simulink model "BBBC_6"  (R2022b)
settings: Solver=VariableStepAuto  StartTime=0.0  StopTime=5  RelTol=1e-3
undefined symbols (not defined in the file): dct, dEv, Ev, sigbuilder_block
libraries: spsMosfetLib x4, spsSeriesRLCBranchLib x4, spsCurrentMeasurementLib x2, spsVoltageMeasurementLib x2, spsGroundLib x1, spsControlledVoltageSourceLib x1, simulink x1, spspowerguiLib x1
settings Model: Creator=Dopechuro  LastModifiedBy=Dopechuro

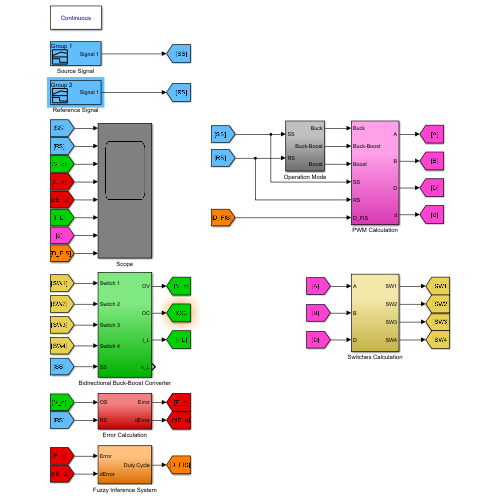
[thumbnail: Simulink's stored preview of the top-level diagram]
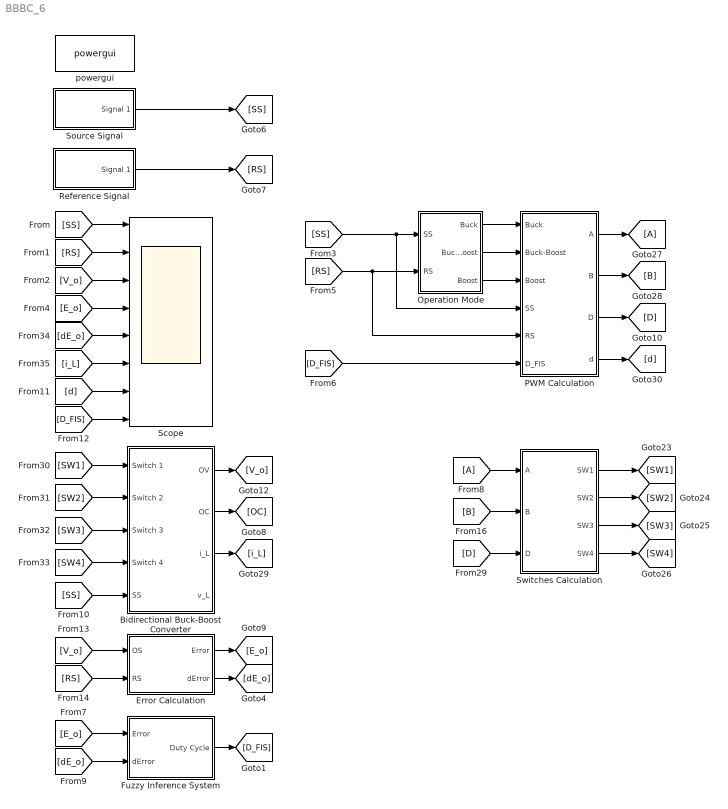
== system BBBC_6 ==
  Bidirectional Buck-Boost Converter : Subsystem
  Error Calculation : Subsystem
  From8 : From
  Fuzzy Inference System : Subsystem
  Goto27 : Goto
  Operation Mode : Subsystem
  PWM Calculation : Subsystem
  Reference Signal : Subsystem  Tag=STV Subsys  LoadFcn=sigbuilder_block('load');  StartFcn=sigbuilder_block('start');  StopFcn=sigbuilder_block('stop');  ClipboardFcn=sigbuilder_block('clipboard');  mask(Sigbuilder block){tuvar=[0:10]}
      mask help: Simulink:masks:SigbuilderBlock_MD
      mask init:
      | if ~strcmp(get_param(bdroot(gcbh),'SimulationStatus'),'stopped') tuvar = sigbuilder_block('maskInit'); end
      settings: CopyFcn=sigbuilder_block('copy');  DeleteFcn=sigbuilder_block('delete');  ModelCloseFcn=sigbuilder_block('modelClose');  PreSaveFcn=sigbuilder_block('preSave');  PauseFcn=sigbuilder_block('pause');  ContinueFcn=sigbuilder_block('continue');  NameChangeFcn=sigbuilder_block('namechange');  OpenFcn=sigbuilder_block('open',[530.25 309.75 550.5 399.75 ]);  CloseFcn=sigbuilder_block('close');
      mask Display: plot(0, 0, 100, 100,[2, 2, 32, 32, 2], [68, 8, 8, 68, 68],[32, 2], [38, 38], [32, 19, 2],[53, 60, 44], [32, 17, 17, 2],[16, 16, 31, 31]);txt = getActiveGroup(gcbh);text(2, 100, txt,'verticalAlignment', 'top');
  Scope : Scope  NumInputPorts=8
  Source Signal : Subsystem  Tag=STV Subsys  LoadFcn=sigbuilder_block('load');  StartFcn=sigbuilder_block('start');  StopFcn=sigbuilder_block('stop');  ClipboardFcn=sigbuilder_block('clipboard');  mask(Sigbuilder block){tuvar=[0:10]}
      mask help: Simulink:masks:SigbuilderBlock_MD
      mask init:
      | if ~strcmp(get_param(bdroot(gcbh),'SimulationStatus'),'stopped') tuvar = sigbuilder_block('maskInit'); end
      settings: CopyFcn=sigbuilder_block('copy');  DeleteFcn=sigbuilder_block('delete');  ModelCloseFcn=sigbuilder_block('modelClose');  PreSaveFcn=sigbuilder_block('preSave');  PauseFcn=sigbuilder_block('pause');  ContinueFcn=sigbuilder_block('continue');  NameChangeFcn=sigbuilder_block('namechange');  OpenFcn=sigbuilder_block('open',[325.5 242.25 550.5 399.75 ]);  CloseFcn=sigbuilder_block('close');
      mask Display: plot(0, 0, 100, 100,[2, 2, 32, 32, 2], [68, 8, 8, 68, 68],[32, 2], [38, 38], [32, 19, 2],[53, 60, 44], [32, 17, 17, 2],[16, 16, 31, 31]);txt = getActiveGroup(gcbh);text(2, 100, txt,'verticalAlignment', 'top');
  Switches Calculation : Subsystem
  powergui : spspowerguiLib/powergui  Priority=1  SimulationMode=Continuous  SampleTime=50e-6  frequency=60  Iterations=50  frequencyindice=0  Pbase=100e6  ErrMax=1e-4  UnitsV=kV  UnitsW=MW  buscounter=0  FunctionMessages=off  echomessages=off  EnableUseOfTLC=off  CurrentSourceSwitches=off  DisableSnubberDevices=off  DisableRonSwitches=off  DisableVfSwitches=off  DisplayEquations=off  AutomaticDiscreteSolvers=off  SolverType=Tustin/Backward Euler (TBE)  Interpol=off  ExternalGateDelay=off  methode=off  Ts=100  x0status=blocks  SPID=on  SwTol=0  HookPort=off  NonlinearTolerance=1e-4  nMaxIteration=100  ContinueOnMaxIteration=off  RestoreLinks=warning  ResistiveCurrentMeasurement=off  Frange=[0:2:500]  Ylog=off  Xlog=on  ShowGrid=off  save=off  variable=ZData  structure=0  ZoomFFT=off  StartTime=0.0  cycles=1  DisplayStyle=1  fundamental=60  FreqAxis=off  MaxFrequency=1000  frequencyindicesteady=1  RmsSteady=1  display=off
  wires:
  [RS] -> Scope/2
  [V_o] -> Scope/3
  [V_o] -> Error Calculation/1(OS)
  [RS] -> Error Calculation/2(RS)
  Error Calculation/1(Error) -> [E_o]
  Error Calculation/2(dError) -> [dE_o]
  [SS] -> Scope/1
  [SS] -> Bidirectional Buck-Boost Converter/5(SS)
  Bidirectional Buck-Boost Converter/1(OV) -> [V_o]
  [E_o] -> Fuzzy Inference System/1(Error)
  [dE_o] -> Fuzzy Inference System/2(dError)
  Fuzzy Inference System/1(Duty Cycle) -> [D_FIS]
  Bidirectional Buck-Boost Converter/2(OC) -> [OC]
  [E_o] -> Scope/4
  [SW1] -> Bidirectional Buck-Boost Converter/1(Switch 1)
  [SW2] -> Bidirectional Buck-Boost Converter/2(Switch 2)
  [SW3] -> Bidirectional Buck-Boost Converter/3(Switch 3)
  [SW4] -> Bidirectional Buck-Boost Converter/4(Switch 4)
  Source Signal/1(Signal 1) -> [SS]
  Reference Signal/1(Signal 1) -> [RS]
  Bidirectional Buck-Boost Converter/3(i_L) -> [i_L]
  [dE_o] -> Scope/5
  [i_L] -> Scope/6
  From8/1 -> Switches Calculation/1(A)
  [B] -> Switches Calculation/2(B)
  [D] -> Switches Calculation/3(D)
  Switches Calculation/1(SW1) -> [SW1]
  Switches Calculation/2(SW2) -> [SW2]
  Switches Calculation/3(SW3) -> [SW3]
  Switches Calculation/4(SW4) -> [SW4]
  [RS] -> Operation Mode/2(RS), PWM Calculation/5(RS)
  Operation Mode/1(Buck) -> PWM Calculation/1(Buck)
  Operation Mode/2(Buck-Boost) -> PWM Calculation/2(Buck-Boost)
  Operation Mode/3(Boost) -> PWM Calculation/3(Boost)
  [D_FIS] -> PWM Calculation/6(D_FIS)
  PWM Calculation/3(D) -> [D]
  PWM Calculation/4(d) -> [d]
  PWM Calculation/1(A) -> Goto27/1
  PWM Calculation/2(B) -> [B]
  [d] -> Scope/7
  [D_FIS] -> Scope/8
  [SS] -> PWM Calculation/4(SS), Operation Mode/1(SS)

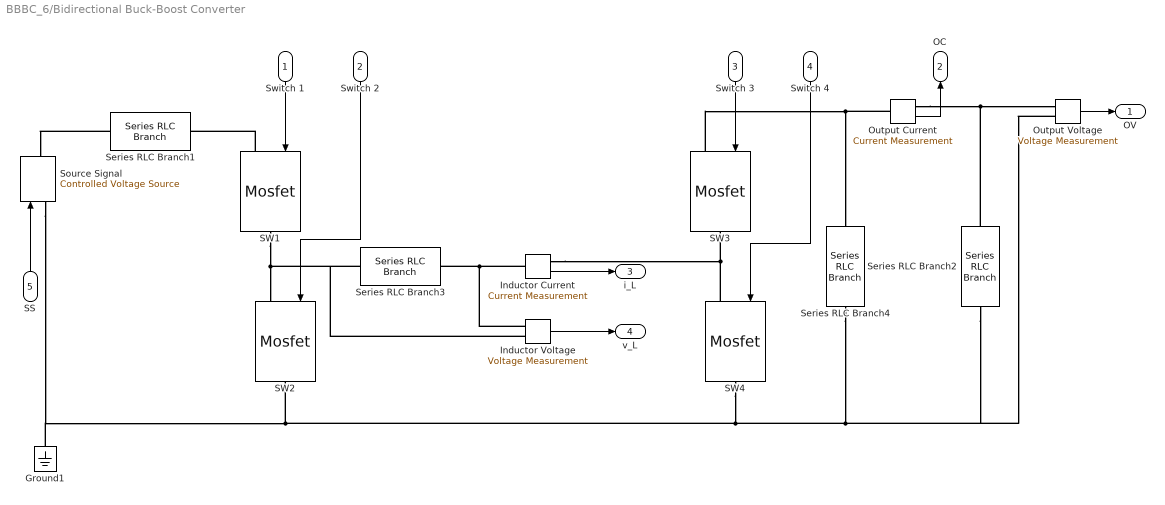
== system BBBC_6/Bidirectional Buck-Boost Converter ==
  Switch 1 : Inport
  Switch 2 : Inport  Port=2
  Switch 3 : Inport  Port=3
  Switch 4 : Inport  Port=4
  SS : Inport  Port=5
  Ground1 : spsGroundLib/Ground  LConnTagsString=a
  Inductor Current : spsCurrentMeasurementLib/Current Measurement  PhasorSimulation=off  OutputType=Complex  PSBequivalent=0
  Inductor Voltage : spsVoltageMeasurementLib/Voltage Measurement  PhasorSimulation=off  OutputType=Complex  PSBequivalent=0
  Output Current : spsCurrentMeasurementLib/Current Measurement  PhasorSimulation=off  OutputType=Complex  PSBequivalent=0
  Output Voltage : spsVoltageMeasurementLib/Voltage Measurement  PhasorSimulation=off  OutputType=Complex  PSBequivalent=0
  SW{1..4} (4 alike) : spsMosfetLib/Mosfet  Ron=0.1  Lon=0  Rd=0.01  Vfd=0  IC=0  Rs=1e5  Cs=inf  Measurements=off
  Series RLC Branch1 : spsSeriesRLCBranchLib/Series RLC Branch  LConnTagsString=__new0  RConnTagsString=__new0  BranchType=R  Resistance=0.1  Inductance=1e-3  SetiL0=off  InitialCurrent=0  Capacitance=1e-6  Setx0=off  InitialVoltage=0  Measurements=None
  Series RLC Branch2 : spsSeriesRLCBranchLib/Series RLC Branch  LConnTagsString=__new0  RConnTagsString=__new0  BranchType=R  Resistance=24  Inductance=1e-3  SetiL0=off  InitialCurrent=0  Capacitance=1000e-6  Setx0=off  InitialVoltage=0  Measurements=None
  Series RLC Branch3 : spsSeriesRLCBranchLib/Series RLC Branch  LConnTagsString=__new0  RConnTagsString=__new0  BranchType=RL  Resistance=0.1  Inductance=0.434e-3  SetiL0=off  InitialCurrent=0  Capacitance=1e-6  Setx0=off  InitialVoltage=0  Measurements=None
  Series RLC Branch4 : spsSeriesRLCBranchLib/Series RLC Branch  LConnTagsString=__new0  RConnTagsString=__new0  BranchType=RC  Resistance=0.01  Inductance=1e-3  SetiL0=off  InitialCurrent=0  Capacitance=10.6e-6  Setx0=off  InitialVoltage=0  Measurements=None
  Source Signal : spsControlledVoltageSourceLib/Controlled Voltage Source  Initialize=off  Source_Type=DC  Amplitude=0  Phase=0  Frequency=0  Measurements=None
  OV : Outport
  OC : Outport  Port=2
  i_L : Outport  Port=3
  v_L : Outport  Port=4
  wires:
  Switch 1/1 -> SW1/1
  Switch 3/1 -> SW3/1
  Switch 2/1 -> SW2/1
  SS/1 -> Source Signal/1
  Switch 4/1 -> SW4/1
  Inductor Current/1 -> i_L/1
  Output Voltage/1 -> OV/1
  Inductor Voltage/1 -> v_L/1
  Output Current/1 -> OC/1
  connections:
  SW1/LConn1 -- Series RLC Branch1/RConn1
  Inductor Current/LConn1 -- Inductor Voltage/LConn2 -- Series RLC Branch3/RConn1
  SW4/LConn1 -- Inductor Current/RConn1 -- SW3/RConn1
  SW4/RConn1 -- Output Voltage/LConn2 -- Series RLC Branch2/RConn1 -- Series RLC Branch4/RConn1 -- Source Signal/LConn1 -- Ground1/LConn1 -- SW2/RConn1
  SW1/RConn1 -- Inductor Voltage/LConn1 -- Series RLC Branch3/LConn1 -- SW2/LConn1
  Series RLC Branch1/LConn1 -- Source Signal/RConn1
  Output Current/RConn1 -- Output Voltage/LConn1 -- Series RLC Branch2/LConn1
  SW3/LConn1 -- Output Current/LConn1 -- Series RLC Branch4/LConn1

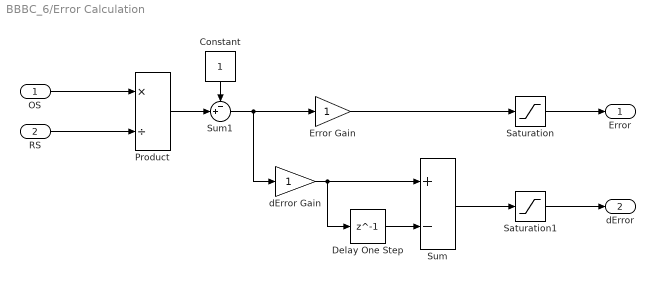
== system BBBC_6/Error Calculation ==
  OS : Inport
  RS : Inport  Port=2
  Constant : Constant
  Delay One Step : Delay  DelayLength=1
  Error Gain : Gain
  Product : Product  Inputs=*/
  Saturation : Saturate  UpperLimit=1  LowerLimit=-1
  Saturation1 : Saturate  UpperLimit=1  LowerLimit=-1
  Sum : Sum  Inputs=+-
  Sum1 : Sum  Inputs=-+|
  dError Gain : Gain
  Error : Outport
  dError : Outport  Port=2
  wires:
  Sum1/1 -> dError Gain/1, Error Gain/1
  dError Gain/1 -> Sum/1, Delay One Step/1
  Error Gain/1 -> Saturation/1
  Constant/1 -> Sum1/1
  Delay One Step/1 -> Sum/2
  Product/1 -> Sum1/2
  Sum/1 -> Saturation1/1
  OS/1 -> Product/1
  RS/1 -> Product/2
  Saturation/1 -> Error/1
  Saturation1/1 -> dError/1

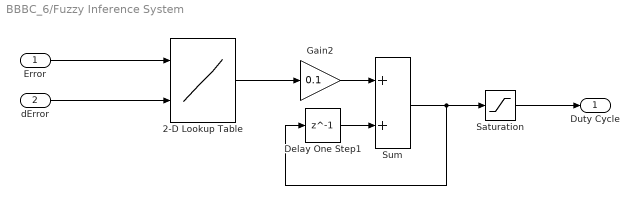
== system BBBC_6/Fuzzy Inference System ==
  Error : Inport
  dError : Inport  Port=2
  2-D Lookup Table : Lookup_n-D  LookupTableObject=''  BreakpointsForDimension1=Ev  BreakpointsForDimension2=dEv  BreakpointsForDimension1FirstPoint=10  BreakpointsForDimension2FirstPoint=10  BreakpointsForDimension1Spacing=12  BreakpointsForDimension2Spacing=12  IndexSearchMethod=Evenly spaced points  Table=dct  InterpMethod=Nearest  DiagnosticForOutOfRangeInput=Warning  InternalRulePriority=Speed  OutDataTypeStr=Inherit: Inherit from 'Table data'  RndMeth=Simplest
      settings: InputPortMap=u0,u1
  Delay One Step1 : Delay  DelayLength=1
  Gain2 : Gain  Gain=0.1
  Saturation : Saturate  UpperLimit=0.9  LowerLimit=-0.9
  Sum : Sum
  Duty Cycle : Outport
  wires:
  Delay One Step1/1 -> Sum/2
  Sum/1 -> Saturation/1, Delay One Step1/1
  Gain2/1 -> Sum/1
  2-D Lookup Table/1 -> Gain2/1
  Saturation/1 -> Duty Cycle/1
  Error/1 -> 2-D Lookup Table/1
  dError/1 -> 2-D Lookup Table/2

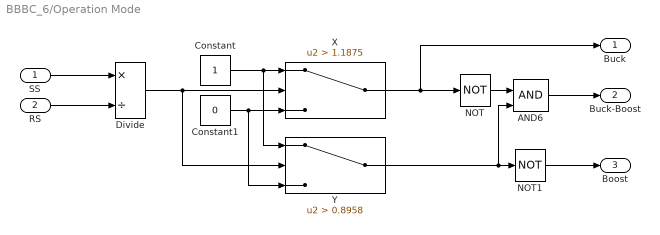
== system BBBC_6/Operation Mode ==
  SS : Inport
  RS : Inport  Port=2
  AND6 : Logic  IconShape=distinctive  AllPortsSameDT=off  OutDataTypeStr=boolean
  Constant : Constant
  Constant1 : Constant  Value=0
  Divide : Product  Inputs=*/
  NOT : Logic  Operator=NOT  IconShape=distinctive  AllPortsSameDT=off  OutDataTypeStr=boolean
  NOT1 : Logic  Operator=NOT  IconShape=distinctive  AllPortsSameDT=off  OutDataTypeStr=boolean
  X : Switch  Criteria=u2 > Threshold  Threshold=1.1875  SaturateOnIntegerOverflow=off  InputSameDT=off
  Y : Switch  Criteria=u2 > Threshold  Threshold=0.8958  SaturateOnIntegerOverflow=off  InputSameDT=off
  Buck : Outport
  Buck-Boost : Outport  Port=2
  Boost : Outport  Port=3
  wires:
  RS/1 -> Divide/2
  Constant/1 -> Y/1, X/1
  Divide/1 -> Y/2, X/2
  X/1 -> Buck/1, NOT/1
  NOT/1 -> AND6/1
  Constant1/1 -> Y/3, X/3
  Y/1 -> NOT1/1, AND6/2
  SS/1 -> Divide/1
  AND6/1 -> Buck-Boost/1
  NOT1/1 -> Boost/1

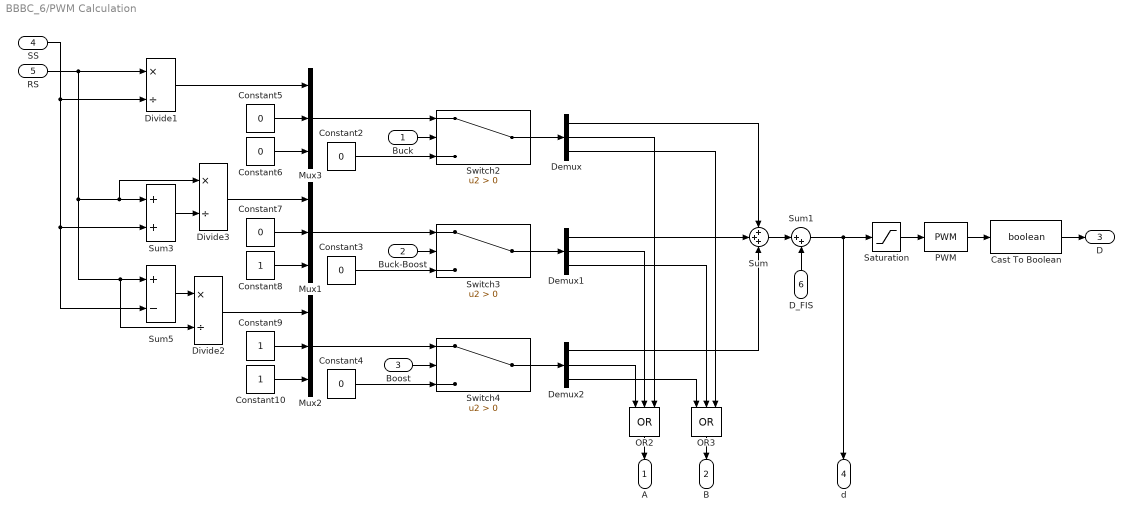
== system BBBC_6/PWM Calculation ==
  Buck : Inport
  Buck-Boost : Inport  Port=2
  Boost : Inport  Port=3
  SS : Inport  Port=4
  RS : Inport  Port=5
  D_FIS : Inport  Port=6
  Cast To Boolean : DataTypeConversion  OutDataTypeStr=boolean  SaturateOnIntegerOverflow=off  RndMeth=Floor
  Constant10 : Constant
  Constant{2..7} (6 alike) : Constant  Value=0
  Constant8 : Constant
  Constant9 : Constant
  Demux : Demux  Outputs=3
  Demux1 : Demux  Outputs=3
  Demux2 : Demux  Outputs=3
  Divide1 : Product  Inputs=*/
  Divide2 : Product  Inputs=*/
  Divide3 : Product  Inputs=*/
  Mux1 : Mux  Inputs=3
  Mux2 : Mux  Inputs=3
  Mux3 : Mux  Inputs=3
  OR2 : Logic  Operator=OR  Inputs=3  IconShape=distinctive  AllPortsSameDT=off  OutDataTypeStr=boolean
  OR3 : Logic  Operator=OR  Inputs=3  IconShape=distinctive  AllPortsSameDT=off  OutDataTypeStr=boolean
  PWM : simulink/Discontinuities/PWM  DisableCoverage=on  Period=1e-5  InitialDelay=0  DisallowZeroDutyCycle=off  RunAtFixedTimeIntervals=off  SampleTime=0.1
  Saturation : Saturate  UpperLimit=0.85  LowerLimit=0.1
  Sum : Sum  Inputs=+++
  Sum1 : Sum  Inputs=|++
  Sum3 : Sum
  Sum5 : Sum  Inputs=+-
  Switch2 : Switch  Criteria=u2 > Threshold  SaturateOnIntegerOverflow=off  InputSameDT=off
  Switch3 : Switch  Criteria=u2 > Threshold  SaturateOnIntegerOverflow=off  InputSameDT=off
  Switch4 : Switch  Criteria=u2 > Threshold  SaturateOnIntegerOverflow=off  InputSameDT=off
  A : Outport
  B : Outport  Port=2
  D : Outport  Port=3
  d : Outport  Port=4
  wires:
  Constant6/1 -> Mux3/3
  Constant2/1 -> Switch2/3
  Switch4/1 -> Demux2/1
  Sum3/1 -> Divide3/2
  Constant5/1 -> Mux3/2
  Mux3/1 -> Switch2/1
  Sum1/1 -> Saturation/1, d/1
  Constant8/1 -> Mux1/3
  Demux1/1 -> Sum/2
  D_FIS/1 -> Sum1/2
  Sum/1 -> Sum1/1
  Switch3/1 -> Demux1/1
  Switch2/1 -> Demux/1
  Constant4/1 -> Switch4/3
  Demux/3 -> OR3/3
  Buck-Boost/1 -> Switch3/2
  Demux2/1 -> Sum/3
  Demux2/2 -> OR2/1
  Sum5/1 -> Divide2/1
  RS/1 -> Divide1/1, Sum3/1, Divide3/1, Sum5/1, Divide2/2
  Divide1/1 -> Mux3/1
  Demux/2 -> OR2/3
  Demux2/3 -> OR3/1
  Cast To Boolean/1 -> D/1
  Demux1/2 -> OR2/2
  Constant10/1 -> Mux2/3
  Demux/1 -> Sum/1
  OR3/1 -> B/1
  Mux2/1 -> Switch4/1
  PWM/1 -> Cast To Boolean/1
  Demux1/3 -> OR3/2
  Constant3/1 -> Switch3/3
  SS/1 -> Divide1/2, Sum3/2, Sum5/2
  Divide2/1 -> Mux2/1
  Mux1/1 -> Switch3/1
  Constant9/1 -> Mux2/2
  Constant7/1 -> Mux1/2
  Divide3/1 -> Mux1/1
  OR2/1 -> A/1
  Boost/1 -> Switch4/2
  Buck/1 -> Switch2/2
  Saturation/1 -> PWM/1

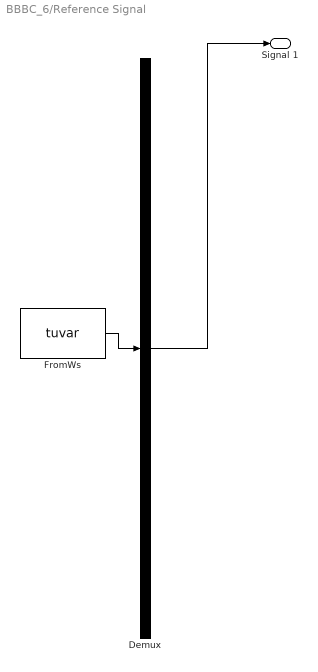
== system BBBC_6/Reference Signal ==
  Demux : Demux  Tag=STV Demux  Outputs=1
      settings: DisplayOption=none
  FromWs : FromWorkspace  Tag=STV FromWs  VariableName=tuvar
      SigBuilderData=|
      | common.afterFinalStr = 'Extrapolate'
      | common.sampleTime = 0
      | dataSet.timeRange = [0 5]
      | dataSet.name = 'Group 2'
      | sbobj.Groups.Name = 'Group 2'
      | sbobj.Groups.Signals.Name = 'Signal 1'
      | sbobj.Groups.Signals.XData = [0 5]
      | sbobj.Groups.Signals.YData = [48 48]
      | sbobj.Groups.TimeRange = [0 5]
  Signal 1 : Outport  Tag=STV Outport
  wires:
  FromWs/1 -> Demux/1
  Demux/1 -> Signal 1/1

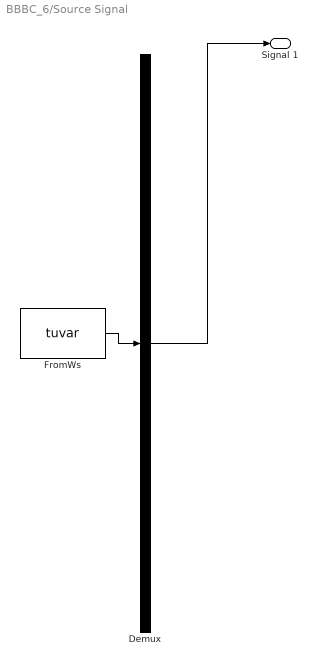
== system BBBC_6/Source Signal ==
  Demux : Demux  Tag=STV Demux  Outputs=1
      settings: DisplayOption=none
  FromWs : FromWorkspace  Tag=STV FromWs  VariableName=tuvar
      SigBuilderData=|
      | common.afterFinalStr = 'Extrapolate'
      | common.sampleTime = 0
      | dataSet.timeRange = [0 5]
      | dataSet.name = 'Group 1'
      | sbobj.Groups.Name = 'Group 1'
      | sbobj.Groups.Signals.Name = 'Signal 1'
      | sbobj.Groups.Signals.XData = [0 5]
      | sbobj.Groups.Signals.YData = [70 35]
      | sbobj.Groups.TimeRange = [0 5]
  Signal 1 : Outport  Tag=STV Outport
  wires:
  FromWs/1 -> Demux/1
  Demux/1 -> Signal 1/1

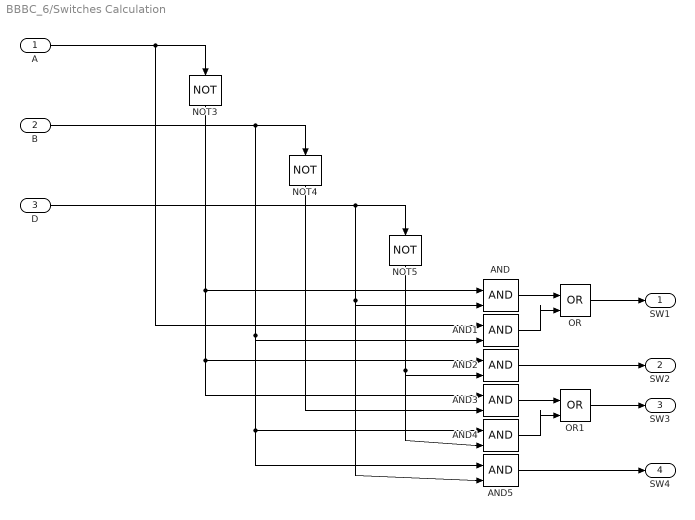
== system BBBC_6/Switches Calculation ==
  A : Inport
  B : Inport  Port=2
  D : Inport  Port=3
  AND{,1..5} (6 alike) : Logic  IconShape=distinctive  AllPortsSameDT=off  OutDataTypeStr=boolean
  NOT3 : Logic  Operator=NOT  IconShape=distinctive  AllPortsSameDT=off  OutDataTypeStr=boolean
  NOT4 : Logic  Operator=NOT  IconShape=distinctive  AllPortsSameDT=off  OutDataTypeStr=boolean
  NOT5 : Logic  Operator=NOT  IconShape=distinctive  AllPortsSameDT=off  OutDataTypeStr=boolean
  OR : Logic  Operator=OR  IconShape=distinctive  AllPortsSameDT=off  OutDataTypeStr=boolean
  OR1 : Logic  Operator=OR  IconShape=distinctive  AllPortsSameDT=off  OutDataTypeStr=boolean
  SW1 : Outport
  SW2 : Outport  Port=2
  SW3 : Outport  Port=3
  SW4 : Outport  Port=4
  wires:
  NOT5/1 -> AND4/2, AND2/2
  B/1 -> AND1/2, AND4/1, AND5/1, NOT4/1
  A/1 -> AND1/1, NOT3/1
  D/1 -> NOT5/1, AND5/2, AND/2
  NOT3/1 -> AND/1, AND2/1, AND3/1
  AND1/1 -> OR/2
  NOT4/1 -> AND3/2
  AND2/1 -> SW2/1
  AND4/1 -> OR1/2
  AND/1 -> OR/1
  AND3/1 -> OR1/1
  OR1/1 -> SW3/1
  OR/1 -> SW1/1
  AND5/1 -> SW4/1
